simulink library "LumMiscBlockset"  (R2015b)
settings: Solver=ode45  StartTime=0.0  StopTime=10.0  RelTol=1e-3
settings Model: Creator=Christopher  LastModifiedBy=Christopher
settings DataIOCC: SaveFormat=Array
settings DebuggingCC: SolverPrmCheckMsg=warning
settings HardwareCC: ProdBitPerPointer=32  ProdLargestAtomicFloat=None  ProdIntDivRoundTo=Undefined  ProdEndianess=Unspecified  ProdWordSize=32  ProdHWDeviceType=32-bit Generic
settings GRTTargetCC: GeneratePreprocessorConditionals=Disable all
settings ConfigComp: CovModelRefEnable=Off  CovSFcnEnable=off

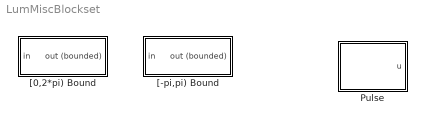
== system LumMiscBlockset ==
  Pulse : Subsystem  mask{pulse_time=0, pulse_duration=1, pulse_amplitude=1}
      mask prompts: pulse_time "Start time (sec)"; pulse_duration "Duration (sec)"; pulse_amplitude "Amplitude"
      mask help:
      | Create a single pulse.
      |
      | INPUT:  None
      |
      | OUTPUT: pulse of the specified duration and magnitude.
      |
      | Created by Christopher Lum
      | lum@u.washington.edu
  "[-pi,pi) Bound" : Subsystem  Description=|
      | Version History  
      |                  
      | 05/??/05: Created
      mask help:
      | Converts input angle to it equivalent in the range [-pi,pi).
      |
      | Inputs:		In: input angle (rad)
      | Outputs:	Out (bounded): bounded angle in range [-pi,pi).
      |
      | Created by Christopher Lum
      | lum@u.washington.edu
      |
      | Original Block concept from Aerosim Blockset by Unmanned Dynamics.  www.u-dynamics.com
  "[0,2*pi) Bound" : Subsystem  Description=|
      | Version History  
      |                  
      | 05/??/05: Created
      mask help:
      | Converts input angle to it equivalent in the range [0,2*pi).
      |
      | Inputs:		In: input angle (rad)
      | Outputs:	Out (bounded): bounded angle in range [0,2*pi).
      |
      | Created by Christopher Lum
      | lum@u.washington.edu
      |
      | Original Block concept from Aerosim Blockset by Unmanned Dynamics.  www.u-dynamics.com

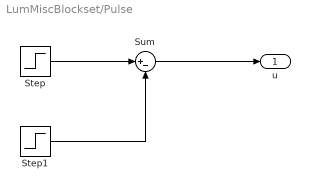
== system LumMiscBlockset/Pulse ==
  Step : Step  Time=pulse_time  After=pulse_amplitude  SampleTime=0
  Step1 : Step  Time=pulse_time + pulse_duration  After=pulse_amplitude  SampleTime=0
  Sum : Sum  Inputs=|+-
  u : Outport
  wires:
  Step/1 -> Sum/1
  Step1/1 -> Sum/2
  Sum/1 -> u/1

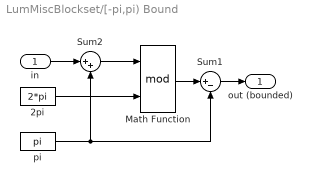
== system LumMiscBlockset/[-pi,pi) Bound ==
  in : Inport
  2pi : Constant  Value=2*pi
  Math Function : Math  Operator=mod  SaturateOnIntegerOverflow=on
  Sum1 : Sum  Inputs=|+-  SaturateOnIntegerOverflow=on  InputSameDT=on  OutDataTypeStr=Inherit: Same as first input
  Sum2 : Sum  Inputs=|++  SaturateOnIntegerOverflow=on  InputSameDT=on  OutDataTypeStr=Inherit: Same as first input
  pi : Constant  Value=pi
  out (bounded) : Outport
  wires:
  Math Function/1 -> Sum1/1
  2pi/1 -> Math Function/2
  Sum2/1 -> Math Function/1
  pi/1 -> Sum2/2, Sum1/2
  in/1 -> Sum2/1
  Sum1/1 -> out (bounded)/1

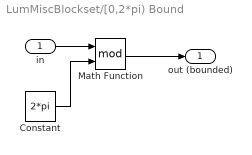
== system LumMiscBlockset/[0,2*pi) Bound ==
  in : Inport
  Constant : Constant  Value=2*pi
  Math Function : Math  Operator=mod  SaturateOnIntegerOverflow=on
  out (bounded) : Outport
  wires:
  in/1 -> Math Function/1
  Math Function/1 -> out (bounded)/1
  Constant/1 -> Math Function/2
